simulink model "mergedModels"  (R2022a)
settings: Solver=FixedStepAuto  StartTime=0.0  StopTime=10.0  FixedStep=1e-3  RelTol=1e-3  EnableMultiTasking=on
undefined symbols (not defined in the file): D0, D1, D10, D11, D12, D13, D2, D3, D4, D5, D6, D7, D8, D9, PTA0, PTA1, PTA2, PTB23, PTB9, PTC16, PTC17, PTC2, PTC3, PTC4, PTD0, PTD1, PTD2, PTD3
libraries: frdmk64flib x42
settings Model: ExtModeTrigDuration=5  Creator=ethan  LastModifiedBy=gurle
settings OptimizationCC: EnhancedBackFolding=on  PassReuseOutputArgsAs=Individual arguments  ZeroExternalMemoryAtStartup=off  ZeroInternalMemoryAtStartup=off  MaxStackSize=64  OptimizeBlockOrder=speed  DifferentSizesBufferReuse=on  OptimizationCustomize=off  EfficientTunableParamExpr=on
settings DebuggingCC: ParameterTunabilityLossMsg=error
settings HardwareCC: ProdBitPerPointer=32  ProdBitPerSizeT=32  ProdBitPerPtrDiffT=32  ProdLargestAtomicInteger=Long  ProdLargestAtomicFloat=Double  ProdWordSize=32  ProdHWDeviceType=ARM Compatible->ARM Cortex
settings SFSimCC: MATLABDynamicMemAlloc=off
settings RTWCC: SystemTargetFile=ert.tlc  HardwareBoard=NXP FRDM-K64F  TLCOptions="-aInlineSetEventsForThisBaseRateFcn=TLC_FALSE -aSuppressMultiTaskScheduler=TLC_FALSE  -aRateBasedStepFcn=0"  TemplateMakefile=ert_default_tmf  Toolchain=GNU Tools for ARM Embedded Processors
settings CodeAppCC: ForceParamTrailComments=on  IgnoreCustomStorageClasses=off  OperatorAnnotations=on  SimulinkDataObjDesc=on  SFDataObjDesc=on  InsertBlockDesc=on
settings ERTTargetCC: ExtModeTransport=4  ExtModeMexFile=sendToCommService

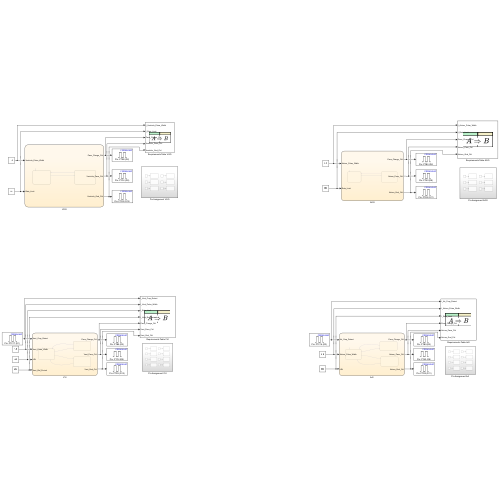
[thumbnail: Simulink's stored preview of the top-level diagram]
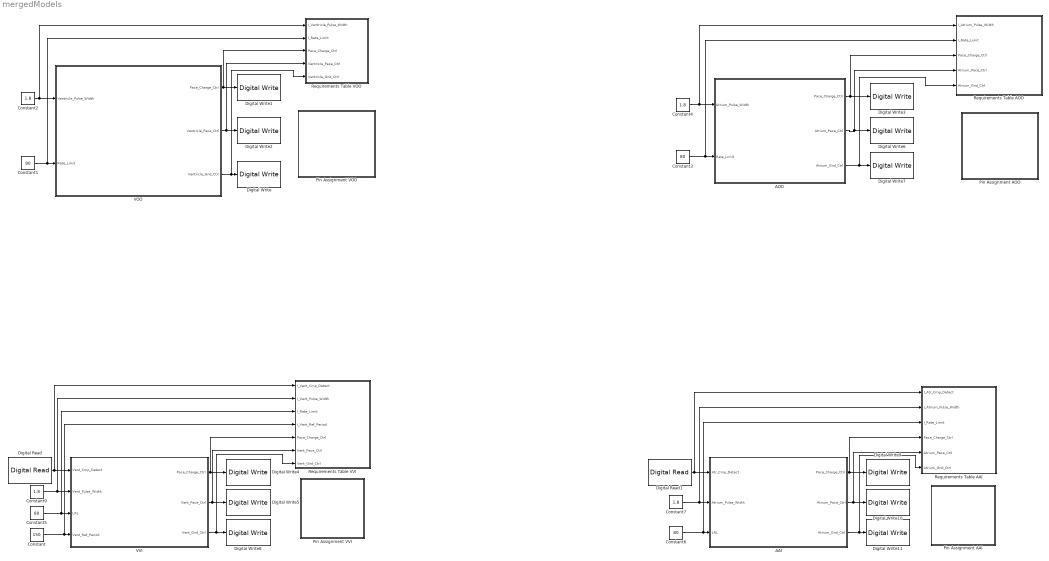
== system mergedModels ==
  AAI : Stateflow chart  TreatAsAtomicUnit=on
  AOO : Stateflow chart  TreatAsAtomicUnit=on
      settings: PortSchema="{\"entries\":[{\"content\":{\"sides\":[{\"content\":{\"connectorIds\":[\"In1\",\"In2\"]},\"type\":\"ConnectorPlacement.EquallySpacedRectSide\",\"uuid\":\"680d5ad3-d091-43dc-b942-9150701a6dd0\"},{\"content\":{\"connectorIds\":[\"Out1\",\"Out3\",\"Out2\"],\"side\":\"RIGHT\"},\"type\":\"ConnectorPlacement.EquallySpacedRectSide\",\"uuid\":\"5c4ab46d-119d-425a-a6f0-c11b7d896570\"},{\"content\":{\"connectorIds\":[],\"side\":\"TOP\"},\"type\":\"ConnectorPlacement.EquallySpacedRectSide\",\"uuid\":\"0b6eb296-b2d5-496b-a1dc-abb07009583a\"}]},\"type\":\"ConnectorPlacement.EquallySpacedConnector\",\"uuid\":\"b5598554-2186-446c-b16e-60380e5c7438\"}],\"packageUris\":[\"http://schema.mathworks.com/mf0/Connector/R2020b\"],\"version\":\"1.0\"}"
  Constant : Constant  Value=150  OutDataTypeStr=int16
  Constant1 : Constant  Value=80  OutDataTypeStr=double
  Constant{2,4,7,9} (4 alike) : Constant  Value=1.8
  Constant3 : Constant  Value=80  OutDataTypeStr=double
  Constant5 : Constant  Value=80
  Constant6 : Constant  Value=80
  Digital Read : frdmk64flib/Digital Read  Whichpin=PTC17 (D1)  SampleTime=-1
  Digital Read1 : frdmk64flib/Digital Read  Whichpin=PTC16 (D0)  SampleTime=-1
  Digital Write : frdmk64flib/Digital Write  Whichpin=PTD3 (D12)
  Digital Write{1,3..4,9} (4 alike) : frdmk64flib/Digital Write  Whichpin=PTB9 (D2)
  Digital Write10 : frdmk64flib/Digital Write  Whichpin=PTA0 (D8)
  Digital Write11 : frdmk64flib/Digital Write  Whichpin=PTD2 (D11)
  Digital Write2 : frdmk64flib/Digital Write  Whichpin=PTC4 (D9)
  Digital Write5 : frdmk64flib/Digital Write  Whichpin=PTC4 (D9)
  Digital Write6 : frdmk64flib/Digital Write  Whichpin=PTA0 (D8)
  Digital Write7 : frdmk64flib/Digital Write  Whichpin=PTD2 (D11)
  Digital Write8 : frdmk64flib/Digital Write  Whichpin=PTD3 (D12)
  Pin Assignment AAI : Subsystem
  Pin Assignment AOO : Subsystem
  Pin Assignment VOO : Subsystem
  Pin Assignment VVI : Subsystem
  Requirements Table AAI : Requirements Table  TreatAsAtomicUnit=on
  Requirements Table AOO : Requirements Table  TreatAsAtomicUnit=on
  Requirements Table VOO : Requirements Table  TreatAsAtomicUnit=on
  Requirements Table VVI : Requirements Table  TreatAsAtomicUnit=on
  VOO : Stateflow chart  TreatAsAtomicUnit=on
  VVI : Stateflow chart  TreatAsAtomicUnit=on
      settings: PortSchema="{\"entries\":[{\"content\":{\"sides\":[{\"content\":{\"connectorIds\":[\"In1\",\"In2\",\"In4\",\"In3\"]},\"type\":\"ConnectorPlacement.EquallySpacedRectSide\",\"uuid\":\"77befb9f-4f07-4a71-b7f1-2c262bc1904d\"},{\"content\":{\"connectorIds\":[\"Out1\",\"Out2\",\"Out3\"],\"side\":\"RIGHT\"},\"type\":\"ConnectorPlacement.EquallySpacedRectSide\",\"uuid\":\"0e23ffc0-fff8-4b52-b26b-28bd9c2ea1c8\"},{\"content\":{\"connectorIds\":[],\"side\":\"TOP\"},\"type\":\"ConnectorPlacement.EquallySpacedRectSide\",\"uuid\":\"4490f046-066c-4589-a3d2-d91c8e90418c\"}]},\"type\":\"ConnectorPlacement.EquallySpacedConnector\",\"uuid\":\"c0d430be-3514-4a93-9359-fa603ef3c0f0\"}],\"packageUris\":[\"http://schema.mathworks.com/mf0/Connector/R2020b\"],\"version\":\"1.0\"}"
  wires:
  AAI/3(Atrium_Gnd_Ctrl) -> Requirements Table AAI/6(Atrium_Gnd_Ctrl), Digital Write11/1
  Constant6/1 -> Requirements Table AAI/3(I_Rate_Limit), AAI/3(LRL)
  Constant7/1 -> AAI/2(Atrium_Pulse_Width), Requirements Table AAI/2(I_Atrium_Pulse_Width)
  AAI/2(Atrium_Pace_Ctrl) -> Digital Write10/1, Requirements Table AAI/5(Atrium_Pace_Ctrl)
  Digital Read1/1 -> AAI/1(Atr_Cmp_Detect), Requirements Table AAI/1(I_Atr_Cmp_Detect)
  AAI/1(Pace_Charge_Ctrl) -> Digital Write9/1, Requirements Table AAI/4(Pace_Charge_Ctrl)
  AOO/2(Atrium_Gnd_Ctrl) -> Digital Write7/1, Requirements Table AOO/5(Atrium_Gnd_Ctrl)
  AOO/3(Atrium_Pace_Ctrl) -> Digital Write6/1, Requirements Table AOO/4(Atrium_Pace_Ctrl)
  Constant4/1 -> Requirements Table AOO/1(I_Atrium_Pulse_Width), AOO/1(Atrium_Pulse_Width)
  Constant3/1 -> Requirements Table AOO/2(I_Rate_Limit), AOO/2(Rate_Limit)
  AOO/1(Pace_Charge_Ctrl) -> Digital Write3/1, Requirements Table AOO/3(Pace_Charge_Ctrl)
  VOO/2(Ventricle_Pace_Ctrl) -> Digital Write2/1, Requirements Table VOO/4(Ventricle_Pace_Ctrl)
  VOO/3(Ventricle_Gnd_Ctrl) -> Requirements Table VOO/5(Ventricle_Gnd_Ctrl), Digital Write/1
  Constant2/1 -> VOO/1(Ventricle_Pulse_Width), Requirements Table VOO/1(I_Ventricle_Pulse_Width)
  Constant1/1 -> Requirements Table VOO/2(I_Rate_Limit), VOO/2(Rate_Limit)
  VOO/1(Pace_Charge_Ctrl) -> Digital Write1/1, Requirements Table VOO/3(Pace_Charge_Ctrl)
  Digital Read/1 -> VVI/1(Vent_Cmp_Detect), Requirements Table VVI/1(I_Vent_Cmp_Detect)
  Constant/1 -> Requirements Table VVI/4(I_Vent_Ref_Period), VVI/3(Vent_Ref_Period)
  VVI/1(Pace_Charge_Ctrl) -> Digital Write4/1, Requirements Table VVI/5(Pace_Charge_Ctrl)
  Constant9/1 -> VVI/2(Vent_Pulse_Width), Requirements Table VVI/2(I_Vent_Pulse_Width)
  VVI/3(Vent_Gnd_Ctrl) -> Requirements Table VVI/7(Vent_Gnd_Ctrl), Digital Write8/1
  Constant5/1 -> VVI/4(LRL), Requirements Table VVI/3(I_Rate_Limit)
  VVI/2(Vent_Pace_Ctrl) -> Digital Write5/1, Requirements Table VVI/6(Vent_Pace_Ctrl)

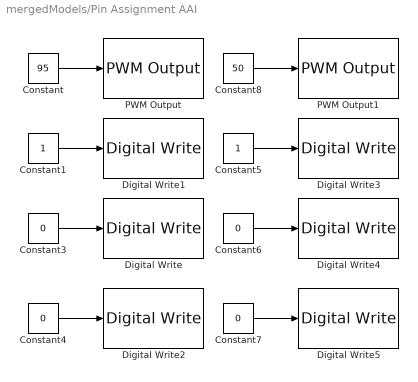
== system mergedModels/Pin Assignment AAI ==
  Constant : Constant  Value=95  OutDataTypeStr=int8
  Constant1 : Constant
  Constant{3..4,6..7} (4 alike) : Constant  Value=0
  Constant5 : Constant
  Constant8 : Constant  Value=50  OutDataTypeStr=int8
  Digital Write : frdmk64flib/Digital Write  Whichpin=PTB23 (D4)
  Digital Write1 : frdmk64flib/Digital Write  Whichpin=PTD1 (D13)
  Digital Write2 : frdmk64flib/Digital Write  Whichpin=PTC3 (D7)
  Digital Write3 : frdmk64flib/Digital Write  Whichpin=PTD0 (D10)
  Digital Write4 : frdmk64flib/Digital Write  Whichpin=PTD3 (D12)
  Digital Write5 : frdmk64flib/Digital Write  Whichpin=PTC4 (D9)
  PWM Output : frdmk64flib/PWM Output  Whichpin=PTC2 (D6)  InitialFrequency=2000  InitialDutyCycle=0
  PWM Output1 : frdmk64flib/PWM Output  Whichpin=PTA2 (D5)  InitialFrequency=2000  InitialDutyCycle=0
  wires:
  Constant1/1 -> Digital Write1/1
  Constant5/1 -> Digital Write3/1
  Constant7/1 -> Digital Write5/1
  Constant4/1 -> Digital Write2/1
  Constant/1 -> PWM Output/1
  Constant8/1 -> PWM Output1/1
  Constant3/1 -> Digital Write/1
  Constant6/1 -> Digital Write4/1

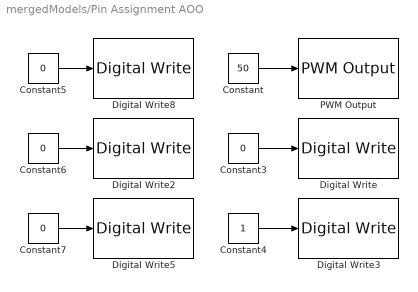
== system mergedModels/Pin Assignment AOO ==
  Constant : Constant  Value=50  OutDataTypeStr=int8
  Constant{3,5..7} (4 alike) : Constant  Value=0  OutDataTypeStr=int8
  Constant4 : Constant  OutDataTypeStr=int8
  Digital Write : frdmk64flib/Digital Write  Whichpin=PTD3 (D12)
  Digital Write2 : frdmk64flib/Digital Write  Whichpin=PTC4 (D9)
  Digital Write3 : frdmk64flib/Digital Write  Whichpin=PTD0 (D10)
  Digital Write5 : frdmk64flib/Digital Write  Whichpin=PTC3 (D7)
  Digital Write8 : frdmk64flib/Digital Write  Whichpin=PTB23 (D4)
  PWM Output : frdmk64flib/PWM Output  Whichpin=PTA2 (D5)  InitialFrequency=2000  InitialDutyCycle=0
  wires:
  Constant4/1 -> Digital Write3/1
  Constant/1 -> PWM Output/1
  Constant7/1 -> Digital Write5/1
  Constant5/1 -> Digital Write8/1
  Constant6/1 -> Digital Write2/1
  Constant3/1 -> Digital Write/1

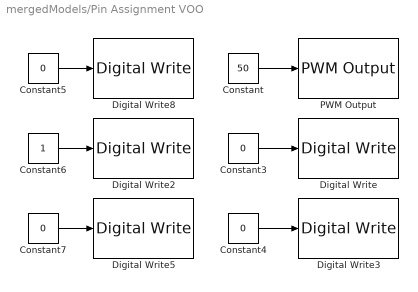
== system mergedModels/Pin Assignment VOO ==
  Constant : Constant  Value=50  OutDataTypeStr=int8
  Constant{3..5,7} (4 alike) : Constant  Value=0  OutDataTypeStr=int8
  Constant6 : Constant  OutDataTypeStr=int8
  Digital Write : frdmk64flib/Digital Write  Whichpin=PTB23 (D4)
  Digital Write2 : frdmk64flib/Digital Write  Whichpin=PTD0 (D10)
  Digital Write3 : frdmk64flib/Digital Write  Whichpin=PTD2 (D11)
  Digital Write5 : frdmk64flib/Digital Write  Whichpin=PTC3 (D7)
  Digital Write8 : frdmk64flib/Digital Write  Whichpin=PTA0 (D8)
  PWM Output : frdmk64flib/PWM Output  Whichpin=PTA2 (D5)  InitialFrequency=2000  InitialDutyCycle=0
  wires:
  Constant4/1 -> Digital Write3/1
  Constant/1 -> PWM Output/1
  Constant7/1 -> Digital Write5/1
  Constant5/1 -> Digital Write8/1
  Constant6/1 -> Digital Write2/1
  Constant3/1 -> Digital Write/1

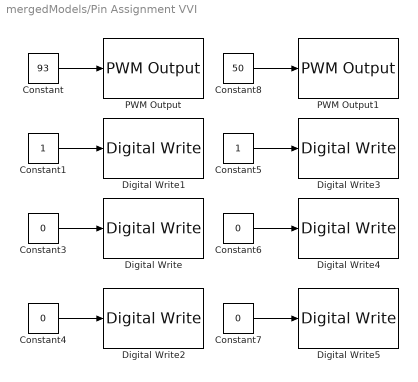
== system mergedModels/Pin Assignment VVI ==
  Constant : Constant  Value=93  OutDataTypeStr=int8
  Constant1 : Constant
  Constant{3..4,6..7} (4 alike) : Constant  Value=0
  Constant5 : Constant
  Constant8 : Constant  Value=50  OutDataTypeStr=int8
  Digital Write : frdmk64flib/Digital Write  Whichpin=PTB23 (D4)
  Digital Write1 : frdmk64flib/Digital Write  Whichpin=PTD1 (D13)
  Digital Write2 : frdmk64flib/Digital Write  Whichpin=PTC3 (D7)
  Digital Write3 : frdmk64flib/Digital Write  Whichpin=PTD0 (D10)
  Digital Write4 : frdmk64flib/Digital Write  Whichpin=PTD2 (D11)
  Digital Write5 : frdmk64flib/Digital Write  Whichpin=PTA0 (D8)
  PWM Output : frdmk64flib/PWM Output  Whichpin=PTA1 (D3)  InitialFrequency=2000  InitialDutyCycle=0
  PWM Output1 : frdmk64flib/PWM Output  Whichpin=PTA2 (D5)  InitialFrequency=2000  InitialDutyCycle=0
  wires:
  Constant1/1 -> Digital Write1/1
  Constant5/1 -> Digital Write3/1
  Constant7/1 -> Digital Write5/1
  Constant4/1 -> Digital Write2/1
  Constant/1 -> PWM Output/1
  Constant8/1 -> PWM Output1/1
  Constant3/1 -> Digital Write/1
  Constant6/1 -> Digital Write4/1

== stateflow chart mergedModels/Requirements Table VOO ==
  (default) -> (junction 1073742358)
  (junction 1073742358) -> (junction 1073742359) : {
      | % SF_REQ_REV_07
      | }
  (junction 1073742359) -> (junction 1073742361) : {
      | % HEADER_ASSIGNMENTS
      |
      | }
  (junction 1073742361) -> (junction 1073742363) : {
      | % START_A_4
      | }
  (junction 1073742363) -> (junction 1073742365) : {
      | }
  (junction 1073742365) -> (junction 1073742367)
  (junction 1073742367) -> (junction 1073742369) : {
      | }
  (junction 1073742369) -> (junction 1073742371) : {
      | % END_A_4
      | }
  (junction 1073742371) -> (junction 1073742373) : {
      | % START_R_10
      | }
  (junction 1073742373) -> (junction 1073742375) : {
      | }
  (junction 1073742375) -> (junction 1073742377)
  (junction 1073742377) -> (junction 1073742379) [order 1] : [(((I_Rate_Limit) == (30)) || ((I_Rate_Limit) == (35)) || ((I_Rate_Limit) == (40)) || ((I_Rate_Limit) == (45)) || ((I_Rate_Limit) == (50)) || ((I_Rate_Limit) == (51)) || ((I_Rate_Limit) == (52)) || ((I_Rate_Limit) == (53)) || ((I_Rate_Limit) == (54)) || ((I_Rate_Limit) == (55)) || ((I_Rate_Limit) == (56)) || ((I_Rate_Limit) == (57)) || ((I_Rate_Limit) == (58)) || ((I_Rate_Limit) == (59)) || ((I_Rate_Limit) == (60)) || ((I_Rate_Limit) == (61)) || ((I_Rate_Limit) == (62)) || ((I_Rate_Limit) == (63)) || ((I_Rate_Limit) == (64)) || ((I_Rate_Limit) == (65)) || ((I_Rate_Limit) == (66)) || ((I_Rate_Limit) == (67)) || ((I_Rate_Limit) == (68)) || ((I_Rate_Limit) == (69)) || ((I_Rate_Limit) == (70)) || ((I_Rate_Limit) == (71)) || ((I_Rate_Limit) == (72)) || ((I_Rate_Limit) == (73)) || ((I_Rate_Limit) == (74)) || ((I_Rate_Limit) == (75)) || ((I_Rate_Limit) == (76)) || ((I_Rate_Limit) == (77)) || ((I_Rate_Limit) == (78)) || ((I_Rate_Limit) == (79)) || ((I_Rate_Limit) == (80)) || ((I_Rate_Limit) == (81)) || ((I_Rate_Limit) == (82)) || ((I_Rate_Limit) == (83)) || ((I_Rate_Limit) == (84)) || ((I_Rate_Limit) == (85)) || ((I_Rate_Limit) == (86)) || ((I_Rate_Limit) == (87)) || ((I_Rate_Limit) == (88)) || ((I_Rate_Limit) == (89)) || ((I_Rate_Limit) == (90)) || ((I_Rate_Limit) == (95)) || ((I_Rate_Limit) == (100)) || ((I_Rate_Limit) == (105)) || ((I_Rate_Limit) == (110)) || ((I_Rate_Limit) == (115)) || ((I_Rate_Limit) == (120)) || ((I_Rate_Limit) == (125)) || ((I_Rate_Limit) == (130)) || ((I_Rate_Limit) == (135)) || ((I_Rate_Limit) == (140)) || ((I_Rate_Limit) == (145)) || ((I_Rate_Limit) == (150)) || ((I_Rate_Limit) == (155)) || ((I_Rate_Limit) == (160)) || ((I_Rate_Limit) == (165)) || ((I_Rate_Limit) == (170)) || ((I_Rate_Limit) == (175))) && (((I_Ventricle_Pulse_Width) == (0.05)) || ((I_Ventricle_Pulse_Width) == (0.1)) || ((I_Ventricle_Pulse_Width) == (0.2)) || ((I_Ventricle_Pulse_Width) == (0.3)) || ((I_Ventricle_Pulse_Width) == (0.4)) || ((I_Ventricle_Pulse_Width) == (0.5)) || ((I_Ventricle_Pulse_Width) == (0.6)) || ((I_Ventricle_Pulse_Width) == (0.7)) || ((I_Ventricle_Pulse_Width) == (0.8)) || ((I_Ventricle_Pulse_Width) == (0.9)) || ((I_Ventricle_Pulse_Width) == (1)) || ((I_Ventricle_Pulse_Width) == (1.1)) || ((I_Ventricle_Pulse_Width) == (1.2)) || ((I_Ventricle_Pulse_Width) == (1.3)) || ((I_Ventricle_Pulse_Width) == (1.4)) || ((I_Ventricle_Pulse_Width) == (1.5)) || ((I_Ventricle_Pulse_Width) == (1.6)) || ((I_Ventricle_Pulse_Width) == (1.7)) || ((I_Ventricle_Pulse_Width) == (1.8)) || ((I_Ventricle_Pulse_Width) == (1.9)))]
  (junction 1073742377) -> (junction 1073742385) [order 2]
  (junction 1073742379) -> (junction 1073742381) : {
      | reqtable_postcondition(((Pace_Charge_Ctrl == true && Ventricle_Gnd_Ctrl == true && Ventricle_Pace_Ctrl == false) || (Pace_Charge_Ctrl == false && Ventricle_Gnd_Ctrl == false && Ventricle_Pace_Ctrl == true)), 'R:1');
      |
      |
      | }
  (junction 1073742381) -> (junction 1073742383) : {
      | }
  (junction 1073742383) -> (junction 1073742385)
  (junction 1073742385) -> (junction 1073742387)
  (junction 1073742387) -> (junction 1073742389) : {
      | % END_R_10
      | }
  data: I_Ventricle_Pulse_Width input; I_Rate_Limit input; Pace_Charge_Ctrl input; Ventricle_Pace_Ctrl input; Ventricle_Gnd_Ctrl input

== stateflow chart mergedModels/AOO ==
  state Charge_C22
    entry:
    Atrium_Pace_Ctrl = false;
    Atrium_Gnd_Ctrl = true;
    Pace_Charge_Ctrl = true;
  state Discharge_C22
    entry:
    Pace_Charge_Ctrl = false;
    Atrium_Pace_Ctrl = true;
    Atrium_Gnd_Ctrl = false;
  (default) -> Charge_C22
  Discharge_C22 -> Charge_C22 : after(Atrium_Pulse_Width,msec)
  Charge_C22 -> Discharge_C22 : after((60000/Rate_Limit)-Atrium_Pulse_Width,msec)
  data: Pace_Charge_Ctrl output; Atrium_Gnd_Ctrl output; Atrium_Pace_Ctrl output; Atrium_Pulse_Width input; Rate_Limit input

== stateflow chart mergedModels/VOO ==
  state Charge_C22
    entry:
    Ventricle_Pace_Ctrl = false;
    Ventricle_Gnd_Ctrl = true;
    Pace_Charge_Ctrl = true;
  state Discharge_C22
    entry:
    Pace_Charge_Ctrl = false;
    Ventricle_Gnd_Ctrl = false;
    Ventricle_Pace_Ctrl = true;
  (default) -> Charge_C22
  Discharge_C22 -> Charge_C22 : after(Ventricle_Pulse_Width,msec)
  Charge_C22 -> Discharge_C22 : after((60000/Rate_Limit)-Ventricle_Pulse_Width,msec)
  data: Pace_Charge_Ctrl output; Ventricle_Pace_Ctrl output; Ventricle_Gnd_Ctrl output; Ventricle_Pulse_Width input; Rate_Limit input

== stateflow chart mergedModels/Requirements Table AOO ==
  (default) -> (junction 1073741860)
  (junction 1073741860) -> (junction 1073741861) : {
      | % SF_REQ_REV_07
      | }
  (junction 1073741861) -> (junction 1073741863) : {
      | % HEADER_ASSIGNMENTS
      |
      | }
  (junction 1073741863) -> (junction 1073741865) : {
      | % START_A_4
      | }
  (junction 1073741865) -> (junction 1073741867) : {
      | }
  (junction 1073741867) -> (junction 1073741869)
  (junction 1073741869) -> (junction 1073741871) : {
      | }
  (junction 1073741871) -> (junction 1073741873) : {
      | % END_A_4
      | }
  (junction 1073741873) -> (junction 1073741915) : {
      | % START_R_1
      | }
  (junction 1073741915) -> (junction 1073741917) : {
      | }
  (junction 1073741917) -> (junction 1073741919)
  (junction 1073741919) -> (junction 1073741921) [order 1] : [(((I_Rate_Limit) == (30)) || ((I_Rate_Limit) == (35)) || ((I_Rate_Limit) == (40)) || ((I_Rate_Limit) == (45)) || ((I_Rate_Limit) == (50)) || ((I_Rate_Limit) == (51)) || ((I_Rate_Limit) == (52)) || ((I_Rate_Limit) == (53)) || ((I_Rate_Limit) == (54)) || ((I_Rate_Limit) == (55)) || ((I_Rate_Limit) == (56)) || ((I_Rate_Limit) == (57)) || ((I_Rate_Limit) == (58)) || ((I_Rate_Limit) == (59)) || ((I_Rate_Limit) == (60)) || ((I_Rate_Limit) == (61)) || ((I_Rate_Limit) == (62)) || ((I_Rate_Limit) == (63)) || ((I_Rate_Limit) == (64)) || ((I_Rate_Limit) == (65)) || ((I_Rate_Limit) == (66)) || ((I_Rate_Limit) == (67)) || ((I_Rate_Limit) == (68)) || ((I_Rate_Limit) == (69)) || ((I_Rate_Limit) == (70)) || ((I_Rate_Limit) == (71)) || ((I_Rate_Limit) == (72)) || ((I_Rate_Limit) == (73)) || ((I_Rate_Limit) == (74)) || ((I_Rate_Limit) == (75)) || ((I_Rate_Limit) == (76)) || ((I_Rate_Limit) == (77)) || ((I_Rate_Limit) == (78)) || ((I_Rate_Limit) == (79)) || ((I_Rate_Limit) == (80)) || ((I_Rate_Limit) == (81)) || ((I_Rate_Limit) == (82)) || ((I_Rate_Limit) == (83)) || ((I_Rate_Limit) == (84)) || ((I_Rate_Limit) == (85)) || ((I_Rate_Limit) == (86)) || ((I_Rate_Limit) == (87)) || ((I_Rate_Limit) == (88)) || ((I_Rate_Limit) == (89)) || ((I_Rate_Limit) == (90)) || ((I_Rate_Limit) == (95)) || ((I_Rate_Limit) == (100)) || ((I_Rate_Limit) == (105)) || ((I_Rate_Limit) == (110)) || ((I_Rate_Limit) == (115)) || ((I_Rate_Limit) == (120)) || ((I_Rate_Limit) == (125)) || ((I_Rate_Limit) == (130)) || ((I_Rate_Limit) == (135)) || ((I_Rate_Limit) == (140)) || ((I_Rate_Limit) == (145)) || ((I_Rate_Limit) == (150)) || ((I_Rate_Limit) == (155)) || ((I_Rate_Limit) == (160)) || ((I_Rate_Limit) == (165)) || ((I_Rate_Limit) == (170)) || ((I_Rate_Limit) == (175))) && (((I_Atrium_Pulse_Width) == (0.05)) || ((I_Atrium_Pulse_Width) == (0.1)) || ((I_Atrium_Pulse_Width) == (0.2)) || ((I_Atrium_Pulse_Width) == (0.3)) || ((I_Atrium_Pulse_Width) == (0.4)) || ((I_Atrium_Pulse_Width) == (0.5)) || ((I_Atrium_Pulse_Width) == (0.6)) || ((I_Atrium_Pulse_Width) == (0.7)) || ((I_Atrium_Pulse_Width) == (0.8)) || ((I_Atrium_Pulse_Width) == (0.9)) || ((I_Atrium_Pulse_Width) == (1)) || ((I_Atrium_Pulse_Width) == (1.1)) || ((I_Atrium_Pulse_Width) == (1.2)) || ((I_Atrium_Pulse_Width) == (1.3)) || ((I_Atrium_Pulse_Width) == (1.4)) || ((I_Atrium_Pulse_Width) == (1.5)) || ((I_Atrium_Pulse_Width) == (1.6)) || ((I_Atrium_Pulse_Width) == (1.7)) || ((I_Atrium_Pulse_Width) == (1.8)) || ((I_Atrium_Pulse_Width) == (1.9)))]
  (junction 1073741919) -> (junction 1073741927) [order 2]
  (junction 1073741921) -> (junction 1073741923) : {
      | reqtable_postcondition(((Pace_Charge_Ctrl == true && Atrium_Gnd_Ctrl == true && Atrium_Pace_Ctrl == false) || (Pace_Charge_Ctrl == false && Atrium_Gnd_Ctrl == false && Atrium_Pace_Ctrl == true)), 'R:1');
      |
      |
      | }
  (junction 1073741923) -> (junction 1073741925) : {
      | }
  (junction 1073741925) -> (junction 1073741927)
  (junction 1073741927) -> (junction 1073741929)
  (junction 1073741929) -> (junction 1073741931) : {
      | % END_R_1
      | }
  data: I_Atrium_Pulse_Width input; I_Rate_Limit input; Pace_Charge_Ctrl input; Atrium_Pace_Ctrl input; Atrium_Gnd_Ctrl input

== stateflow chart mergedModels/Requirements Table VVI ==
  (default) -> (junction 1073742126)
  (junction 1073742126) -> (junction 1073742127) : {
      | % SF_REQ_REV_07
      | }
  (junction 1073742127) -> (junction 1073742129) : {
      | % HEADER_ASSIGNMENTS
      |
      | }
  (junction 1073742129) -> (junction 1073742131) : {
      | % START_A_4
      | }
  (junction 1073742131) -> (junction 1073742133) : {
      | }
  (junction 1073742133) -> (junction 1073742135)
  (junction 1073742135) -> (junction 1073742137) : {
      | }
  (junction 1073742137) -> (junction 1073742139) : {
      | % END_A_4
      | }
  (junction 1073742139) -> (junction 1073742212) : {
      | % START_R_10
      | }
  (junction 1073742212) -> (junction 1073742214) : {
      | }
  (junction 1073742214) -> (junction 1073742216)
  (junction 1073742216) -> (junction 1073742218) [order 1] : [(((I_Vent_Pulse_Width) == (0.05)) || ((I_Vent_Pulse_Width) == (0.1)) || ((I_Vent_Pulse_Width) == (0.2)) || ((I_Vent_Pulse_Width) == (0.3)) || ((I_Vent_Pulse_Width) == (0.4)) || ((I_Vent_Pulse_Width) == (0.5)) || ((I_Vent_Pulse_Width) == (0.6)) || ((I_Vent_Pulse_Width) == (0.7)) || ((I_Vent_Pulse_Width) == (0.8)) || ((I_Vent_Pulse_Width) == (0.9)) || ((I_Vent_Pulse_Width) == (1)) || ((I_Vent_Pulse_Width) == (1.1)) || ((I_Vent_Pulse_Width) == (1.2)) || ((I_Vent_Pulse_Width) == (1.3)) || ((I_Vent_Pulse_Width) == (1.4)) || ((I_Vent_Pulse_Width) == (1.5)) || ((I_Vent_Pulse_Width) == (1.6)) || ((I_Vent_Pulse_Width) == (1.7)) || ((I_Vent_Pulse_Width) == (1.8)) || ((I_Vent_Pulse_Width) == (1.9)) || ((I_Vent_Pulse_Width) == (20))) && (((I_Rate_Limit) == (30)) || ((I_Rate_Limit) == (35)) || ((I_Rate_Limit) == (40)) || ((I_Rate_Limit) == (45)) || ((I_Rate_Limit) == (50)) || ((I_Rate_Limit) == (51)) || ((I_Rate_Limit) == (52)) || ((I_Rate_Limit) == (53)) || ((I_Rate_Limit) == (54)) || ((I_Rate_Limit) == (55)) || ((I_Rate_Limit) == (56)) || ((I_Rate_Limit) == (57)) || ((I_Rate_Limit) == (58)) || ((I_Rate_Limit) == (59)) || ((I_Rate_Limit) == (60)) || ((I_Rate_Limit) == (61)) || ((I_Rate_Limit) == (62)) || ((I_Rate_Limit) == (63)) || ((I_Rate_Limit) == (64)) || ((I_Rate_Limit) == (65)) || ((I_Rate_Limit) == (66)) || ((I_Rate_Limit) == (67)) || ((I_Rate_Limit) == (68)) || ((I_Rate_Limit) == (69)) || ((I_Rate_Limit) == (70)) || ((I_Rate_Limit) == (71)) || ((I_Rate_Limit) == (72)) || ((I_Rate_Limit) == (73)) || ((I_Rate_Limit) == (74)) || ((I_Rate_Limit) == (75)) || ((I_Rate_Limit) == (76)) || ((I_Rate_Limit) == (77)) || ((I_Rate_Limit) == (78)) || ((I_Rate_Limit) == (79)) || ((I_Rate_Limit) == (80)) || ((I_Rate_Limit) == (81)) || ((I_Rate_Limit) == (82)) || ((I_Rate_Limit) == (83)) || ((I_Rate_Limit) == (84)) || ((I_Rate_Limit) == (85)) || ((I_Rate_Limit) == (86)) || ((I_Rate_Limit) == (87)) || ((I_Rate_Limit) == (88)) || ((I_Rate_Limit) == (89)) || ((I_Rate_Limit) == (90)) || ((I_Rate_Limit) == (95)) || ((I_Rate_Limit) == (100)) || ((I_Rate_Limit) == (105)) || ((I_Rate_Limit) == (110)) || ((I_Rate_Limit) == (115)) || ((I_Rate_Limit) == (120)) || ((I_Rate_Limit) == (125)) || ((I_Rate_Limit) == (130)) || ((I_Rate_Limit) == (135)) || ((I_Rate_Limit) == (140)) || ((I_Rate_Limit) == (145)) || ((I_Rate_Limit) == (150)) || ((I_Rate_Limit) == (155)) || ((I_Rate_Limit) == (160)) || ((I_Rate_Limit) == (165)) || ((I_Rate_Limit) == (170)) || ((I_Rate_Limit) == (175))) && (((I_Vent_Ref_Period) == (150)) || ((I_Vent_Ref_Period) == (160)) || ((I_Vent_Ref_Period) == (170)) || ((I_Vent_Ref_Period) == (180)) || ((I_Vent_Ref_Period) == (190)) || ((I_Vent_Ref_Period) == (200)) || ((I_Vent_Ref_Period) == (210)) || ((I_Vent_Ref_Period) == (220)) || ((I_Vent_Ref_Period) == (230)) || ((I_Vent_Ref_Period) == (240)) || ((I_Vent_Ref_Period) == (250)) || ((I_Vent_Ref_Period) == (260)) || ((I_Vent_Ref_Period) == (270)) || ((I_Vent_Ref_Period) == (280)) || ((I_Vent_Ref_Period) == (290)) || ((I_Vent_Ref_Period) == (300)) || ((I_Vent_Ref_Period) == (310)) || ((I_Vent_Ref_Period) == (320)) || ((I_Vent_Ref_Period) == (330)) || ((I_Vent_Ref_Period) == (340)) || ((I_Vent_Ref_Period) == (350)) || ((I_Vent_Ref_Period) == (360)) || ((I_Vent_Ref_Period) == (370)) || ((I_Vent_Ref_Period) == (380)) || ((I_Vent_Ref_Period) == (390)) || ((I_Vent_Ref_Period) == (400)) || ((I_Vent_Ref_Period) == (410)) || ((I_Vent_Ref_Period) == (420)) || ((I_Vent_Ref_Period) == (430)) || ((I_Vent_Ref_Period) == (440)) || ((I_Vent_Ref_Period) == (450)) || ((I_Vent_Ref_Period) == (460)) || ((I_Vent_Ref_Period) == (470)) || ((I_Vent_Ref_Period) == (480)) || ((I_Vent_Ref_Period) == (490)) || ((I_Vent_Ref_Period) == (500))) && (((I_Vent_Cmp_Detect) == (true)))]
  (junction 1073742216) -> (junction 1073742224) [order 2]
  (junction 1073742218) -> (junction 1073742220) : {
      | reqtable_postcondition(((Pace_Charge_Ctrl == true && Vent_Gnd_Ctrl == true && Vent_Pace_Ctrl == false)), 'R:1');
      |
      |
      | }
  (junction 1073742220) -> (junction 1073742222) : {
      | }
  (junction 1073742222) -> (junction 1073742224)
  (junction 1073742224) -> (junction 1073742226)
  (junction 1073742226) -> (junction 1073742228) : {
      | % END_R_10
      | }
  (junction 1073742228) -> (junction 1073742191) : {
      | % START_R_1
      | }
  (junction 1073742191) -> (junction 1073742193) : {
      | }
  (junction 1073742193) -> (junction 1073742195)
  (junction 1073742195) -> (junction 1073742197) [order 1] : [(((I_Vent_Pulse_Width) == (0.05)) || ((I_Vent_Pulse_Width) == (0.1)) || ((I_Vent_Pulse_Width) == (0.2)) || ((I_Vent_Pulse_Width) == (0.3)) || ((I_Vent_Pulse_Width) == (0.4)) || ((I_Vent_Pulse_Width) == (0.5)) || ((I_Vent_Pulse_Width) == (0.6)) || ((I_Vent_Pulse_Width) == (0.7)) || ((I_Vent_Pulse_Width) == (0.8)) || ((I_Vent_Pulse_Width) == (0.9)) || ((I_Vent_Pulse_Width) == (1)) || ((I_Vent_Pulse_Width) == (1.1)) || ((I_Vent_Pulse_Width) == (1.2)) || ((I_Vent_Pulse_Width) == (1.3)) || ((I_Vent_Pulse_Width) == (1.4)) || ((I_Vent_Pulse_Width) == (1.5)) || ((I_Vent_Pulse_Width) == (1.6)) || ((I_Vent_Pulse_Width) == (1.7)) || ((I_Vent_Pulse_Width) == (1.8)) || ((I_Vent_Pulse_Width) == (1.9))) && (((I_Rate_Limit) == (30)) || ((I_Rate_Limit) == (35)) || ((I_Rate_Limit) == (40)) || ((I_Rate_Limit) == (45)) || ((I_Rate_Limit) == (50)) || ((I_Rate_Limit) == (51)) || ((I_Rate_Limit) == (52)) || ((I_Rate_Limit) == (53)) || ((I_Rate_Limit) == (54)) || ((I_Rate_Limit) == (55)) || ((I_Rate_Limit) == (56)) || ((I_Rate_Limit) == (57)) || ((I_Rate_Limit) == (58)) || ((I_Rate_Limit) == (59)) || ((I_Rate_Limit) == (60)) || ((I_Rate_Limit) == (61)) || ((I_Rate_Limit) == (62)) || ((I_Rate_Limit) == (63)) || ((I_Rate_Limit) == (64)) || ((I_Rate_Limit) == (65)) || ((I_Rate_Limit) == (66)) || ((I_Rate_Limit) == (67)) || ((I_Rate_Limit) == (68)) || ((I_Rate_Limit) == (69)) || ((I_Rate_Limit) == (70)) || ((I_Rate_Limit) == (71)) || ((I_Rate_Limit) == (72)) || ((I_Rate_Limit) == (73)) || ((I_Rate_Limit) == (74)) || ((I_Rate_Limit) == (75)) || ((I_Rate_Limit) == (76)) || ((I_Rate_Limit) == (77)) || ((I_Rate_Limit) == (78)) || ((I_Rate_Limit) == (79)) || ((I_Rate_Limit) == (80)) || ((I_Rate_Limit) == (81)) || ((I_Rate_Limit) == (82)) || ((I_Rate_Limit) == (83)) || ((I_Rate_Limit) == (84)) || ((I_Rate_Limit) == (85)) || ((I_Rate_Limit) == (86)) || ((I_Rate_Limit) == (87)) || ((I_Rate_Limit) == (88)) || ((I_Rate_Limit) == (89)) || ((I_Rate_Limit) == (90)) || ((I_Rate_Limit) == (95)) || ((I_Rate_Limit) == (100)) || ((I_Rate_Limit) == (105)) || ((I_Rate_Limit) == (110)) || ((I_Rate_Limit) == (115)) || ((I_Rate_Limit) == (120)) || ((I_Rate_Limit) == (125)) || ((I_Rate_Limit) == (130)) || ((I_Rate_Limit) == (135)) || ((I_Rate_Limit) == (140)) || ((I_Rate_Limit) == (145)) || ((I_Rate_Limit) == (150)) || ((I_Rate_Limit) == (155)) || ((I_Rate_Limit) == (160)) || ((I_Rate_Limit) == (165)) || ((I_Rate_Limit) == (170)) || ((I_Rate_Limit) == (175))) && (((I_Vent_Ref_Period) == (150)) || ((I_Vent_Ref_Period) == (160)) || ((I_Vent_Ref_Period) == (170)) || ((I_Vent_Ref_Period) == (180)) || ((I_Vent_Ref_Period) == (190)) || ((I_Vent_Ref_Period) == (200)) || ((I_Vent_Ref_Period) == (210)) || ((I_Vent_Ref_Period) == (220)) || ((I_Vent_Ref_Period) == (230)) || ((I_Vent_Ref_Period) == (240)) || ((I_Vent_Ref_Period) == (250)) || ((I_Vent_Ref_Period) == (260)) || ((I_Vent_Ref_Period) == (270)) || ((I_Vent_Ref_Period) == (280)) || ((I_Vent_Ref_Period) == (290)) || ((I_Vent_Ref_Period) == (300)) || ((I_Vent_Ref_Period) == (310)) || ((I_Vent_Ref_Period) == (320)) || ((I_Vent_Ref_Period) == (330)) || ((I_Vent_Ref_Period) == (340)) || ((I_Vent_Ref_Period) == (350)) || ((I_Vent_Ref_Period) == (360)) || ((I_Vent_Ref_Period) == (370)) || ((I_Vent_Ref_Period) == (380)) || ((I_Vent_Ref_Period) == (390)) || ((I_Vent_Ref_Period) == (400)) || ((I_Vent_Ref_Period) == (410)) || ((I_Vent_Ref_Period) == (420)) || ((I_Vent_Ref_Period) == (430)) || ((I_Vent_Ref_Period) == (440)) || ((I_Vent_Ref_Period) == (450)) || ((I_Vent_Ref_Period) == (460)) || ((I_Vent_Ref_Period) == (470)) || ((I_Vent_Ref_Period) == (480)) || ((I_Vent_Ref_Period) == (490)) || ((I_Vent_Ref_Period) == (500))) && (((I_Vent_Cmp_Detect) == (false)))]
  (junction 1073742195) -> (junction 1073742203) [order 2]
  (junction 1073742197) -> (junction 1073742199) : {
      | reqtable_postcondition(((Pace_Charge_Ctrl == true && Vent_Gnd_Ctrl == true && Vent_Pace_Ctrl == false) || (Pace_Charge_Ctrl == false && Vent_Gnd_Ctrl == false && Vent_Pace_Ctrl == true)), 'R:2');
      |
      |
      | }
  (junction 1073742199) -> (junction 1073742201) : {
      | }
  (junction 1073742201) -> (junction 1073742203)
  (junction 1073742203) -> (junction 1073742205)
  (junction 1073742205) -> (junction 1073742207) : {
      | % END_R_1
      | }
  data: I_Vent_Cmp_Detect input; I_Vent_Pulse_Width input; I_Rate_Limit input; I_Vent_Ref_Period input; Pace_Charge_Ctrl input; Vent_Pace_Ctrl input; Vent_Gnd_Ctrl input

== stateflow chart mergedModels/VVI ==
  state Inhibit
    entry:
    Vent_Pace_Ctrl = false;
    Vent_Gnd_Ctrl = true;
    Pace_Charge_Ctrl = true;
  state Signal_Search
    entry:
    Vent_Pace_Ctrl = false;
    Vent_Gnd_Ctrl = true;
    Pace_Charge_Ctrl = true;
  state Pace
    entry:
    Pace_Charge_Ctrl = false;
    Vent_Pace_Ctrl = true;
    Vent_Gnd_Ctrl = false;
  Inhibit -> Signal_Search : after(Vent_Ref_Period,msec)
  (default) -> Signal_Search
  Signal_Search -> Inhibit [order 2] : [Vent_Cmp_Detect == true]
  Signal_Search -> Pace [order 1] : [after(((60000/LRL)-Vent_Pulse_Width),msec)]
  Pace -> Signal_Search : after(Vent_Pulse_Width,msec)
  data: Vent_Cmp_Detect input boolean; Vent_Pulse_Width input; Vent_Ref_Period input; Pace_Charge_Ctrl output; Vent_Pace_Ctrl output; Vent_Gnd_Ctrl output; LRL input

== stateflow chart mergedModels/AAI ==
  state Inhibit
    entry:
    Atrium_Pace_Ctrl = false;
    Atrium_Gnd_Ctrl = true;
    Pace_Charge_Ctrl = true;
  state Signal_Search
    entry:
    Atrium_Pace_Ctrl = false;
    Atrium_Gnd_Ctrl = true;
    Pace_Charge_Ctrl = true;
  state Pace
    entry:
    Pace_Charge_Ctrl = false;
    Atrium_Pace_Ctrl = true;
    Atrium_Gnd_Ctrl = false;
  Inhibit -> Signal_Search : after(((60000/LRL)-Atrium_Pulse_Width)/2,msec)
  (default) -> Signal_Search
  Signal_Search -> Inhibit [order 2] : [Atr_Cmp_Detect == true]
  Signal_Search -> Pace [order 1] : [after(((60000/LRL)-Atrium_Pulse_Width),msec)]
  Pace -> Signal_Search : after(Atrium_Pulse_Width,msec)
  data: Atr_Cmp_Detect input boolean; Atrium_Pulse_Width input; Pace_Charge_Ctrl output; Atrium_Pace_Ctrl output; Atrium_Gnd_Ctrl output; LRL input

== stateflow chart mergedModels/Requirements Table AAI ==
  (default) -> (junction 1073742126)
  (junction 1073742126) -> (junction 1073742127) : {
      | % SF_REQ_REV_07
      | }
  (junction 1073742127) -> (junction 1073742129) : {
      | % HEADER_ASSIGNMENTS
      |
      | }
  (junction 1073742129) -> (junction 1073742131) : {
      | % START_A_4
      | }
  (junction 1073742131) -> (junction 1073742133) : {
      | }
  (junction 1073742133) -> (junction 1073742135)
  (junction 1073742135) -> (junction 1073742137) : {
      | }
  (junction 1073742137) -> (junction 1073742139) : {
      | % END_A_4
      | }
  (junction 1073742139) -> (junction 1073742212) : {
      | % START_R_10
      | }
  (junction 1073742212) -> (junction 1073742214) : {
      | }
  (junction 1073742214) -> (junction 1073742216)
  (junction 1073742216) -> (junction 1073742218) [order 1] : [(((I_Atrium_Pulse_Width) == (0.05)) || ((I_Atrium_Pulse_Width) == (0.1)) || ((I_Atrium_Pulse_Width) == (0.2)) || ((I_Atrium_Pulse_Width) == (0.3)) || ((I_Atrium_Pulse_Width) == (0.4)) || ((I_Atrium_Pulse_Width) == (0.5)) || ((I_Atrium_Pulse_Width) == (0.6)) || ((I_Atrium_Pulse_Width) == (0.7)) || ((I_Atrium_Pulse_Width) == (0.8)) || ((I_Atrium_Pulse_Width) == (0.9)) || ((I_Atrium_Pulse_Width) == (1)) || ((I_Atrium_Pulse_Width) == (1.1)) || ((I_Atrium_Pulse_Width) == (1.2)) || ((I_Atrium_Pulse_Width) == (1.3)) || ((I_Atrium_Pulse_Width) == (1.4)) || ((I_Atrium_Pulse_Width) == (1.5)) || ((I_Atrium_Pulse_Width) == (1.6)) || ((I_Atrium_Pulse_Width) == (1.7)) || ((I_Atrium_Pulse_Width) == (1.8)) || ((I_Atrium_Pulse_Width) == (1.9)) || ((I_Atrium_Pulse_Width) == (20))) && (((I_Rate_Limit) == (30)) || ((I_Rate_Limit) == (35)) || ((I_Rate_Limit) == (40)) || ((I_Rate_Limit) == (45)) || ((I_Rate_Limit) == (50)) || ((I_Rate_Limit) == (51)) || ((I_Rate_Limit) == (52)) || ((I_Rate_Limit) == (53)) || ((I_Rate_Limit) == (54)) || ((I_Rate_Limit) == (55)) || ((I_Rate_Limit) == (56)) || ((I_Rate_Limit) == (57)) || ((I_Rate_Limit) == (58)) || ((I_Rate_Limit) == (59)) || ((I_Rate_Limit) == (60)) || ((I_Rate_Limit) == (61)) || ((I_Rate_Limit) == (62)) || ((I_Rate_Limit) == (63)) || ((I_Rate_Limit) == (64)) || ((I_Rate_Limit) == (65)) || ((I_Rate_Limit) == (66)) || ((I_Rate_Limit) == (67)) || ((I_Rate_Limit) == (68)) || ((I_Rate_Limit) == (69)) || ((I_Rate_Limit) == (70)) || ((I_Rate_Limit) == (71)) || ((I_Rate_Limit) == (72)) || ((I_Rate_Limit) == (73)) || ((I_Rate_Limit) == (74)) || ((I_Rate_Limit) == (75)) || ((I_Rate_Limit) == (76)) || ((I_Rate_Limit) == (77)) || ((I_Rate_Limit) == (78)) || ((I_Rate_Limit) == (79)) || ((I_Rate_Limit) == (80)) || ((I_Rate_Limit) == (81)) || ((I_Rate_Limit) == (82)) || ((I_Rate_Limit) == (83)) || ((I_Rate_Limit) == (84)) || ((I_Rate_Limit) == (85)) || ((I_Rate_Limit) == (86)) || ((I_Rate_Limit) == (87)) || ((I_Rate_Limit) == (88)) || ((I_Rate_Limit) == (89)) || ((I_Rate_Limit) == (90)) || ((I_Rate_Limit) == (95)) || ((I_Rate_Limit) == (100)) || ((I_Rate_Limit) == (105)) || ((I_Rate_Limit) == (110)) || ((I_Rate_Limit) == (115)) || ((I_Rate_Limit) == (120)) || ((I_Rate_Limit) == (125)) || ((I_Rate_Limit) == (130)) || ((I_Rate_Limit) == (135)) || ((I_Rate_Limit) == (140)) || ((I_Rate_Limit) == (145)) || ((I_Rate_Limit) == (150)) || ((I_Rate_Limit) == (155)) || ((I_Rate_Limit) == (160)) || ((I_Rate_Limit) == (165)) || ((I_Rate_Limit) == (170)) || ((I_Rate_Limit) == (175))) && (((I_Atr_Cmp_Detect) == (true)))]
  (junction 1073742216) -> (junction 1073742224) [order 2]
  (junction 1073742218) -> (junction 1073742220) : {
      | reqtable_postcondition(((Pace_Charge_Ctrl == true && Atrium_Gnd_Ctrl == true && Atrium_Pace_Ctrl == false)), 'R:1');
      |
      |
      | }
  (junction 1073742220) -> (junction 1073742222) : {
      | }
  (junction 1073742222) -> (junction 1073742224)
  (junction 1073742224) -> (junction 1073742226)
  (junction 1073742226) -> (junction 1073742228) : {
      | % END_R_10
      | }
  (junction 1073742228) -> (junction 1073742191) : {
      | % START_R_1
      | }
  (junction 1073742191) -> (junction 1073742193) : {
      | }
  (junction 1073742193) -> (junction 1073742195)
  (junction 1073742195) -> (junction 1073742197) [order 1] : [(((I_Atrium_Pulse_Width) == (0.05)) || ((I_Atrium_Pulse_Width) == (0.1)) || ((I_Atrium_Pulse_Width) == (0.2)) || ((I_Atrium_Pulse_Width) == (0.3)) || ((I_Atrium_Pulse_Width) == (0.4)) || ((I_Atrium_Pulse_Width) == (0.5)) || ((I_Atrium_Pulse_Width) == (0.6)) || ((I_Atrium_Pulse_Width) == (0.7)) || ((I_Atrium_Pulse_Width) == (0.8)) || ((I_Atrium_Pulse_Width) == (0.9)) || ((I_Atrium_Pulse_Width) == (1)) || ((I_Atrium_Pulse_Width) == (1.1)) || ((I_Atrium_Pulse_Width) == (1.2)) || ((I_Atrium_Pulse_Width) == (1.3)) || ((I_Atrium_Pulse_Width) == (1.4)) || ((I_Atrium_Pulse_Width) == (1.5)) || ((I_Atrium_Pulse_Width) == (1.6)) || ((I_Atrium_Pulse_Width) == (1.7)) || ((I_Atrium_Pulse_Width) == (1.8)) || ((I_Atrium_Pulse_Width) == (1.9))) && (((I_Rate_Limit) == (30)) || ((I_Rate_Limit) == (35)) || ((I_Rate_Limit) == (40)) || ((I_Rate_Limit) == (45)) || ((I_Rate_Limit) == (50)) || ((I_Rate_Limit) == (51)) || ((I_Rate_Limit) == (52)) || ((I_Rate_Limit) == (53)) || ((I_Rate_Limit) == (54)) || ((I_Rate_Limit) == (55)) || ((I_Rate_Limit) == (56)) || ((I_Rate_Limit) == (57)) || ((I_Rate_Limit) == (58)) || ((I_Rate_Limit) == (59)) || ((I_Rate_Limit) == (60)) || ((I_Rate_Limit) == (61)) || ((I_Rate_Limit) == (62)) || ((I_Rate_Limit) == (63)) || ((I_Rate_Limit) == (64)) || ((I_Rate_Limit) == (65)) || ((I_Rate_Limit) == (66)) || ((I_Rate_Limit) == (67)) || ((I_Rate_Limit) == (68)) || ((I_Rate_Limit) == (69)) || ((I_Rate_Limit) == (70)) || ((I_Rate_Limit) == (71)) || ((I_Rate_Limit) == (72)) || ((I_Rate_Limit) == (73)) || ((I_Rate_Limit) == (74)) || ((I_Rate_Limit) == (75)) || ((I_Rate_Limit) == (76)) || ((I_Rate_Limit) == (77)) || ((I_Rate_Limit) == (78)) || ((I_Rate_Limit) == (79)) || ((I_Rate_Limit) == (80)) || ((I_Rate_Limit) == (81)) || ((I_Rate_Limit) == (82)) || ((I_Rate_Limit) == (83)) || ((I_Rate_Limit) == (84)) || ((I_Rate_Limit) == (85)) || ((I_Rate_Limit) == (86)) || ((I_Rate_Limit) == (87)) || ((I_Rate_Limit) == (88)) || ((I_Rate_Limit) == (89)) || ((I_Rate_Limit) == (90)) || ((I_Rate_Limit) == (95)) || ((I_Rate_Limit) == (100)) || ((I_Rate_Limit) == (105)) || ((I_Rate_Limit) == (110)) || ((I_Rate_Limit) == (115)) || ((I_Rate_Limit) == (120)) || ((I_Rate_Limit) == (125)) || ((I_Rate_Limit) == (130)) || ((I_Rate_Limit) == (135)) || ((I_Rate_Limit) == (140)) || ((I_Rate_Limit) == (145)) || ((I_Rate_Limit) == (150)) || ((I_Rate_Limit) == (155)) || ((I_Rate_Limit) == (160)) || ((I_Rate_Limit) == (165)) || ((I_Rate_Limit) == (170)) || ((I_Rate_Limit) == (175))) && (((I_Atr_Cmp_Detect) == (false)))]
  (junction 1073742195) -> (junction 1073742203) [order 2]
  (junction 1073742197) -> (junction 1073742199) : {
      | reqtable_postcondition(((Pace_Charge_Ctrl == true && Atrium_Gnd_Ctrl == true && Atrium_Pace_Ctrl == false) || (Pace_Charge_Ctrl == false && Atrium_Gnd_Ctrl == false && Atrium_Pace_Ctrl == true)), 'R:2');
      |
      |
      | }
  (junction 1073742199) -> (junction 1073742201) : {
      | }
  (junction 1073742201) -> (junction 1073742203)
  (junction 1073742203) -> (junction 1073742205)
  (junction 1073742205) -> (junction 1073742207) : {
      | % END_R_1
      | }
  data: I_Atr_Cmp_Detect input; I_Atrium_Pulse_Width input; I_Rate_Limit input; Pace_Charge_Ctrl input; Atrium_Pace_Ctrl input; Atrium_Gnd_Ctrl input
